simulink model "cruise_control_fechada"  (R2020b)
settings: Solver=VariableStepAuto  StartTime=0.0  StopTime=100  RelTol=1e-3
undefined symbols (not defined in the file or in its folder): b, bc, d, Kp, m, vr
settings Model: Creator=mmaximo  LastModifiedBy=kenji

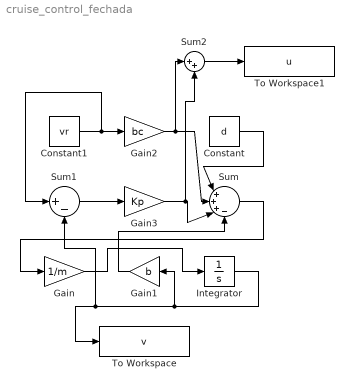
== system cruise_control_fechada ==
  Constant : Constant  Value=d
  Constant1 : Constant  Value=vr
  Gain : Gain  Gain=1/m
  Gain1 : Gain  Gain=b
  Gain2 : Gain  Gain=bc
  Gain3 : Gain  Gain=Kp
  Integrator : Integrator
  Sum : Sum  Inputs=|+++-
  Sum1 : Sum  Inputs=|+-
  Sum2 : Sum  Inputs=|++
  To Workspace : ToWorkspace  VariableName=v  SaveFormat=Structure With Time  SampleTime=-1
  To Workspace1 : ToWorkspace  VariableName=u  SaveFormat=Structure With Time  SampleTime=-1
  wires:
  Constant1/1 -> Sum1/1, Gain2/1
  Sum1/1 -> Gain3/1
  Gain3/1 -> Sum2/2, Sum/3
  Gain2/1 -> Sum2/1, Sum/2
  Constant/1 -> Sum/1
  Sum/1 -> Gain/1
  Gain/1 -> Integrator/1
  Integrator/1 -> Gain1/1, Sum1/2, To Workspace/1
  Gain1/1 -> Sum/4
  Sum2/1 -> To Workspace1/1
